simulink model "qdrdacsim"  (R2012b)
settings: Solver=ode45  StartTime=0.0  StopTime=22000  RelTol=1e-3
values from neighbouring files (symbols this model uses):
  T = 95/2    (= 47.5)    [fluxrampdemodsim.m]
undefined symbols (not defined in the file or in its folder): FRA, FRT, pfb_coeff_gen_calc, sfp, V
libraries: xbsIndex_r4 x5295, casper_library_misc x85, xps_library x14, casper_library_delays x12, maddogLibrary x4, simulink x2
(part 12 of 52)

== system qdrdacsim/syncDelay ==
  sim_1 : Inport
  io_delay : xbsIndex_r4/Delay  rst=off  infoeditControl=Selection of Reset will increase slice count due to use of real FFs and instead of SRLs  en=off  latency=0  dbl_ovrd=off  reg_retiming=on  block_type=delay
  qdrdacsim_syncDelay_user_data_out : xbsIndex_r4/Gateway In  gui_display_data_type=Fixed-point  arith_type=Unsigned  n_bits=32  bin_pt=0  preci_type=Single  exp_width=8  frac_width=24  quantization="Round  (unbiased: +/- Inf)"  overflow=Saturate  period=1  dbl_ovrd=off  timing_constraint=None  locs_specified=off  LOCs={}  UseAsADC=off  ADCChannel='1'  inherit_from_input=off  hdl_port=on  block_type=gatewayin
  reint1 : xbsIndex_r4/Reinterpret  force_arith_type=on  arith_type=Unsigned  force_bin_pt=on  bin_pt=0  block_type=reinterpret
  slice_reg : xbsIndex_r4/Slice  nbits=16  boolean_output=off  mode=Lower Bit Location + Width  bit1=0  base1=MSB of Input  bit0=0  base0=LSB of Input  dbl_ovrd=off  block_type=slice
  in_reg : Outport
  wires:
  qdrdacsim_syncDelay_user_data_out/1 -> io_delay/1
  sim_1/1 -> qdrdacsim_syncDelay_user_data_out/1
  io_delay/1 -> slice_reg/1
  slice_reg/1 -> reint1/1
  reint1/1 -> in_reg/1

== system qdrdacsim/txdestip ==
  sim_1 : Inport
  io_delay : xbsIndex_r4/Delay  rst=off  infoeditControl=Selection of Reset will increase slice count due to use of real FFs and instead of SRLs  en=off  latency=0  dbl_ovrd=off  reg_retiming=on  block_type=delay
  qdrdacsim_txdestip_user_data_out : xbsIndex_r4/Gateway In  gui_display_data_type=Fixed-point  arith_type=Unsigned  n_bits=32  bin_pt=0  preci_type=Single  exp_width=8  frac_width=24  quantization="Round  (unbiased: +/- Inf)"  overflow=Saturate  period=1  dbl_ovrd=off  timing_constraint=None  locs_specified=off  LOCs={}  UseAsADC=off  ADCChannel='1'  inherit_from_input=off  hdl_port=on  block_type=gatewayin
  reint1 : xbsIndex_r4/Reinterpret  force_arith_type=on  arith_type=Unsigned  force_bin_pt=on  bin_pt=0  block_type=reinterpret
  slice_reg : xbsIndex_r4/Slice  nbits=32  boolean_output=off  mode=Lower Bit Location + Width  bit1=0  base1=MSB of Input  bit0=0  base0=LSB of Input  dbl_ovrd=off  block_type=slice
  in_reg : Outport
  wires:
  qdrdacsim_txdestip_user_data_out/1 -> io_delay/1
  sim_1/1 -> qdrdacsim_txdestip_user_data_out/1
  io_delay/1 -> slice_reg/1
  slice_reg/1 -> reint1/1
  reint1/1 -> in_reg/1

== system qdrdacsim/txdestport ==
  sim_1 : Inport
  io_delay : xbsIndex_r4/Delay  rst=off  infoeditControl=Selection of Reset will increase slice count due to use of real FFs and instead of SRLs  en=off  latency=0  dbl_ovrd=off  reg_retiming=on  block_type=delay
  qdrdacsim_txdestport_user_data_out : xbsIndex_r4/Gateway In  gui_display_data_type=Fixed-point  arith_type=Unsigned  n_bits=32  bin_pt=0  preci_type=Single  exp_width=8  frac_width=24  quantization="Round  (unbiased: +/- Inf)"  overflow=Saturate  period=1  dbl_ovrd=off  timing_constraint=None  locs_specified=off  LOCs={}  UseAsADC=off  ADCChannel='1'  inherit_from_input=off  hdl_port=on  block_type=gatewayin
  reint1 : xbsIndex_r4/Reinterpret  force_arith_type=on  arith_type=Unsigned  force_bin_pt=on  bin_pt=0  block_type=reinterpret
  slice_reg : xbsIndex_r4/Slice  nbits=16  boolean_output=off  mode=Lower Bit Location + Width  bit1=0  base1=MSB of Input  bit0=0  base0=LSB of Input  dbl_ovrd=off  block_type=slice
  in_reg : Outport
  wires:
  qdrdacsim_txdestport_user_data_out/1 -> io_delay/1
  sim_1/1 -> qdrdacsim_txdestport_user_data_out/1
  io_delay/1 -> slice_reg/1
  slice_reg/1 -> reint1/1
  reint1/1 -> in_reg/1

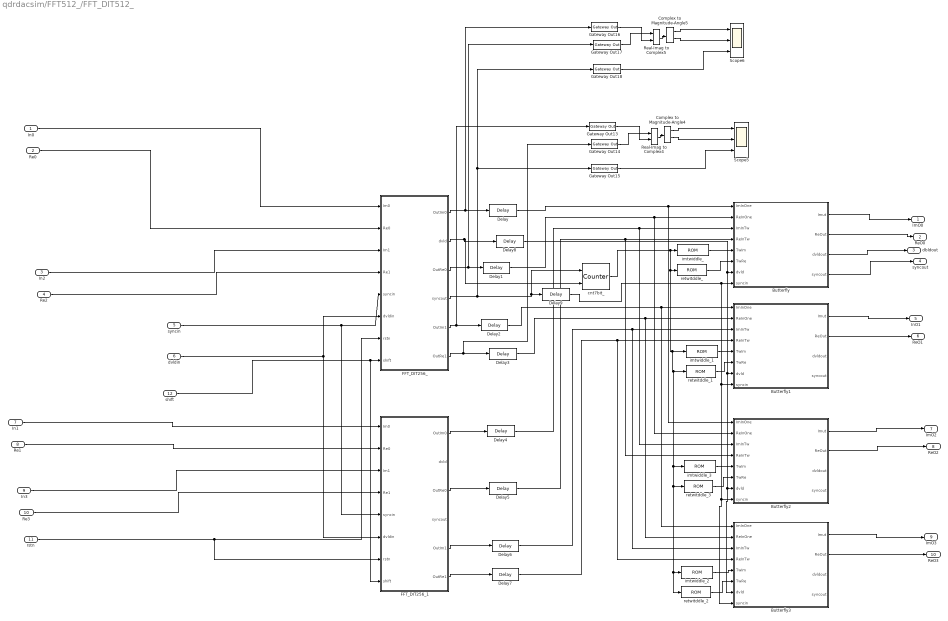
== system qdrdacsim/FFT512_/FFT_DIT512_ ==
  In0 : Inport
  Re0 : Inport  Port=2
  In2 : Inport  Port=3
  Re2 : Inport  Port=4
  syncin : Inport  Port=5
  dvldin : Inport  Port=6
  In1 : Inport  Port=7
  Re1 : Inport  Port=8
  In3 : Inport  Port=9
  Re3 : Inport  Port=10
  rstn : Inport  Port=11
  shift : Inport  Port=12
  Butterfly : Subsystem
  Butterfly1 : Subsystem
  Butterfly2 : Subsystem
  Butterfly3 : Subsystem
  Complex to Magnitude-Angle4 : ComplexToMagnitudeAngle
  Complex to Magnitude-Angle5 : ComplexToMagnitudeAngle
  Delay{,1..9} (10 alike) : xbsIndex_r4/Delay  rst=off  infoeditControl=Selection of Reset will increase slice count due to use of real FFs and instead of SRLs  en=off  latency=1  dbl_ovrd=off  reg_retiming=off  block_type=delay
  FFT_DIT256_ : Subsystem
  FFT_DIT256_1 : Subsystem
  Gateway Out{13..18} (6 alike) : xbsIndex_r4/Gateway Out  inherit_from_input=off  hdl_port=on  timing_constraint=None  locs_specified=off  LOCs={}  UseAsDAC=off  DACChannel='1'  block_type=gatewayout
  Real-Imag to Complex4 : RealImagToComplex
  Real-Imag to Complex5 : RealImagToComplex
  Scope5 : Scope  NumInputPorts=3
      settings: YMin=-5~-5~-5  YMax=5~5~5  SaveName=ScopeData7
  Scope6 : Scope  NumInputPorts=3
      settings: YMin=-5~-5~-5  YMax=5~5~5  SaveName=ScopeData10
  cnt7bit_ : xbsIndex_r4/Counter  cnt_type=Free Running  cnt_to=Inf  operation=Up  start_count=0  cnt_by_val=1  arith_type=Unsigned  n_bits=7  bin_pt=0  load_pin=off  rst=on  en=on  explicit_period=on  period=1  dbl_ovrd=off  use_behavioral_HDL=off  implementation=Fabric  block_type=counter
  imtwiddle_ : xbsIndex_r4/ROM  depth=128  initVector=-sin(2*pi*(0:127)/512)  distributed_mem=Block RAM  rst=off  init_reg=0  en=off  latency=1  gui_display_data_type=Fixed-point  arith_type="Signed  (2's comp)"  n_bits=16  bin_pt=15  preci_type=Single  exp_width=8  frac_width=24  dbl_ovrd=off  optimize=Area  use_rpm=on  block_type=sprom
  imtwiddle_1 : xbsIndex_r4/ROM  depth=128  initVector=-sin(2*pi*(128:255)/512)  distributed_mem=Block RAM  rst=off  init_reg=0  en=off  latency=1  gui_display_data_type=Fixed-point  arith_type="Signed  (2's comp)"  n_bits=16  bin_pt=15  preci_type=Single  exp_width=8  frac_width=24  dbl_ovrd=off  optimize=Area  use_rpm=on  block_type=sprom
  imtwiddle_2 : xbsIndex_r4/ROM  depth=128  initVector=-sin(2*pi*(384:511)/512)  distributed_mem=Block RAM  rst=off  init_reg=0  en=off  latency=1  gui_display_data_type=Fixed-point  arith_type="Signed  (2's comp)"  n_bits=16  bin_pt=15  preci_type=Single  exp_width=8  frac_width=24  dbl_ovrd=off  optimize=Area  use_rpm=on  block_type=sprom
  imtwiddle_3 : xbsIndex_r4/ROM  depth=128  initVector=-sin(2*pi*(256:383)/512)  distributed_mem=Block RAM  rst=off  init_reg=0  en=off  latency=1  gui_display_data_type=Fixed-point  arith_type="Signed  (2's comp)"  n_bits=16  bin_pt=15  preci_type=Single  exp_width=8  frac_width=24  dbl_ovrd=off  optimize=Area  use_rpm=on  block_type=sprom
  retwitddle_ : xbsIndex_r4/ROM  depth=128  initVector=cos(2*pi*(0:127)/512)  distributed_mem=Block RAM  rst=off  init_reg=0  en=off  latency=1  gui_display_data_type=Fixed-point  arith_type="Signed  (2's comp)"  n_bits=16  bin_pt=14  preci_type=Single  exp_width=8  frac_width=24  dbl_ovrd=off  optimize=Area  use_rpm=on  block_type=sprom
  retwitddle_1 : xbsIndex_r4/ROM  depth=128  initVector=cos(2*pi*(128:255)/512)  distributed_mem=Block RAM  rst=off  init_reg=0  en=off  latency=1  gui_display_data_type=Fixed-point  arith_type="Signed  (2's comp)"  n_bits=16  bin_pt=14  preci_type=Single  exp_width=8  frac_width=24  dbl_ovrd=off  optimize=Area  use_rpm=on  block_type=sprom
  retwitddle_2 : xbsIndex_r4/ROM  depth=128  initVector=cos(2*pi*(384:511)/512)  distributed_mem=Block RAM  rst=off  init_reg=0  en=off  latency=1  gui_display_data_type=Fixed-point  arith_type="Signed  (2's comp)"  n_bits=16  bin_pt=14  preci_type=Single  exp_width=8  frac_width=24  dbl_ovrd=off  optimize=Area  use_rpm=on  block_type=sprom
  retwitddle_3 : xbsIndex_r4/ROM  depth=128  initVector=cos(2*pi*(256:383)/512)  distributed_mem=Block RAM  rst=off  init_reg=0  en=off  latency=1  gui_display_data_type=Fixed-point  arith_type="Signed  (2's comp)"  n_bits=16  bin_pt=14  preci_type=Single  exp_width=8  frac_width=24  dbl_ovrd=off  optimize=Area  use_rpm=on  block_type=sprom
  ImO0 : Outport
  ReO0 : Outport  Port=2
  dbldout : Outport  Port=3
  syncout : Outport  Port=4
  InO1 : Outport  Port=5
  ReO1 : Outport  Port=6
  ImO2 : Outport  Port=7
  ReO2 : Outport  Port=8
  ImO3 : Outport  Port=9
  ReO3 : Outport  Port=10
  wires:
  Delay1/1 -> Butterfly2/2(ReInOne), Butterfly/2(ReInOne)
  FFT_DIT256_1/1(OutIm0) -> Delay4/1
  Real-Imag to Complex4/1 -> Complex to Magnitude-Angle4/1
  In1/1 -> FFT_DIT256_1/1(Im0)
  Butterfly1/2(ReOut) -> ReO1/1
  FFT_DIT256_/3(OutRe0) -> Gateway Out17/1, Delay1/1
  FFT_DIT256_/2(dvld) -> Delay8/1, cnt7bit_/2
  Butterfly2/1(Imut) -> ImO2/1
  Complex to Magnitude-Angle5/2 -> Scope6/2
  Delay3/1 -> Butterfly3/2(ReInOne), Butterfly1/2(ReInOne)
  In3/1 -> FFT_DIT256_1/3(Im1)
  retwitddle_1/1 -> Butterfly1/6(TwRe)
  dvldin/1 -> FFT_DIT256_/6(dvldin), FFT_DIT256_1/6(dvldin)
  FFT_DIT256_1/3(OutRe0) -> Delay5/1
  Re3/1 -> FFT_DIT256_1/4(Re1)
  Delay5/1 -> Butterfly2/4(ReInTw), Butterfly/4(ReInTw)
  cnt7bit_/1 -> retwitddle_2/1, imtwiddle_2/1, retwitddle_3/1, imtwiddle_3/1, retwitddle_1/1, imtwiddle_1/1, retwitddle_/1, imtwiddle_/1
  Gateway Out18/1 -> Scope6/3
  Delay6/1 -> Butterfly3/3(ImInTw), Butterfly1/3(ImInTw)
  imtwiddle_2/1 -> Butterfly3/5(TwIm)
  Delay4/1 -> Butterfly2/3(ImInTw), Butterfly/3(ImInTw)
  Gateway Out13/1 -> Real-Imag to Complex4/2
  retwitddle_2/1 -> Butterfly3/6(TwRe)
  Re2/1 -> FFT_DIT256_/4(Re1)
  Gateway Out16/1 -> Real-Imag to Complex5/2
  Re0/1 -> FFT_DIT256_/2(Re0)
  Butterfly/3(dvldout) -> dbldout/1
  Gateway Out17/1 -> Real-Imag to Complex5/1
  Delay/1 -> Butterfly2/1(ImInOne), Butterfly/1(ImInOne)
  Butterfly3/1(Imut) -> ImO3/1
  retwitddle_3/1 -> Butterfly2/6(TwRe)
  imtwiddle_/1 -> Butterfly/5(TwIm)
  imtwiddle_3/1 -> Butterfly2/5(TwIm)
  FFT_DIT256_/1(OutIm0) -> Gateway Out16/1, Delay/1
  Butterfly3/2(ReOut) -> ReO3/1
  Butterfly/1(Imut) -> ImO0/1
  Butterfly/2(ReOut) -> ReO0/1
  FFT_DIT256_1/6(OutRe1) -> Delay7/1
  Delay9/1 -> Butterfly3/8(syncin), Butterfly2/8(syncin), Butterfly1/8(syncin), Butterfly/8(syncin)
  FFT_DIT256_1/5(OutIm1) -> Delay6/1
  Butterfly1/1(Imut) -> InO1/1
  imtwiddle_1/1 -> Butterfly1/5(TwIm)
  Re1/1 -> FFT_DIT256_1/2(Re0)
  Butterfly/4(syncout) -> syncout/1
  FFT_DIT256_/6(OutRe1) -> Gateway Out14/1, Delay3/1
  In0/1 -> FFT_DIT256_/1(Im0)
  Gateway Out14/1 -> Real-Imag to Complex4/1
  Delay7/1 -> Butterfly3/4(ReInTw), Butterfly1/4(ReInTw)
  Butterfly2/2(ReOut) -> ReO2/1
  FFT_DIT256_/4(syncout) -> Gateway Out15/1, Gateway Out18/1, Delay9/1, cnt7bit_/1
  Complex to Magnitude-Angle5/1 -> Scope6/1
  Delay8/1 -> Butterfly3/7(dvld), Butterfly2/7(dvld), Butterfly1/7(dvld), Butterfly/7(dvld)
  FFT_DIT256_/5(OutIm1) -> Gateway Out13/1, Delay2/1
  Real-Imag to Complex5/1 -> Complex to Magnitude-Angle5/1
  retwitddle_/1 -> Butterfly/6(TwRe)
  Complex to Magnitude-Angle4/2 -> Scope5/2
  In2/1 -> FFT_DIT256_/3(Im1)
  Gateway Out15/1 -> Scope5/3
  syncin/1 -> FFT_DIT256_1/5(syncin), FFT_DIT256_/5(syncin)
  Complex to Magnitude-Angle4/1 -> Scope5/1
  Delay2/1 -> Butterfly3/1(ImInOne), Butterfly1/1(ImInOne)
  rstn/1 -> FFT_DIT256_1/7(rstn), FFT_DIT256_/7(rstn)
  shift/1 -> FFT_DIT256_1/8(shift), FFT_DIT256_/8(shift)

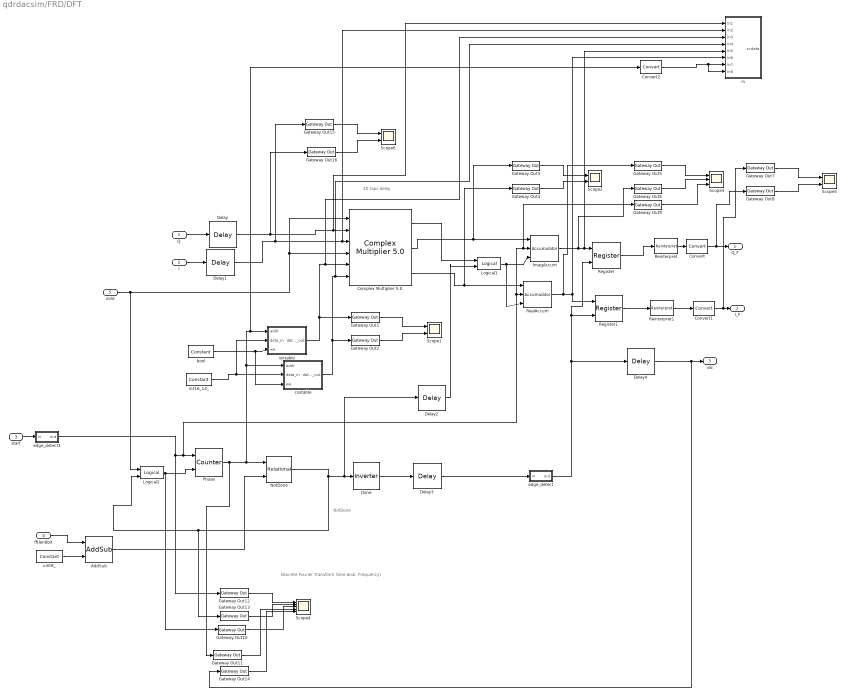
== system qdrdacsim/FRD/DFT ==
  note: 40 taps delay
  note: Discrete Fourier Transform
      | (One Anal. Frequency)
  note: NotDone
  Q : Inport
  I : Inport  Port=2
  start : Inport  Port=3
  fftlen8bit : Inport  Port=4
  dvld : Inport  Port=5
  AddSub : xbsIndex_r4/AddSub  mode=Subtraction  use_carryin=off  use_carryout=off  en=off  latency=0  precision=Full  arith_type=Unsigned  n_bits=16  bin_pt=14  quantization=Truncate  overflow=Wrap  dbl_ovrd=off  use_behavioral_HDL=off  hw_selection=Fabric  pipelined=off  block_type=addsub
  "Complex Multiplier 5.0 " : xbsIndex_r4/Complex Multiplier 5.0   hasatlast=off  hasatuser=off  atuserwidth=1  hasbtlast=off  hasbtuser=off  btuserwidth=1  multtype=Use_Mults  optimizegoal=Resources  flowcontrol=NonBlocking  outputwidth=20  roundmode=Truncate  hasctrltlast=off  hasctrltuser=off  ctrltuserwidth=1  outtlastbehv=Null  latencyconfig=Manual  minimumlatency=40  aclken=off  aresetn=off  trim_axipin_name=on  aportwidth=63  bportwidth=63  ip_name=Complex Multiplier  ip_version=5.0  dsptool_ready=true  ipcore_usecache=true  ipcore_useipmodelcache=true  ipcore_verbose=false  ipcore_latency_parameter='minimumlatency'  wrapper_available=true  port_translation_map={ 'aclken' => 'en', 'aresetn' => 'rst'}  structural_sim=false  block_type=cmpy_v5_0
  Convert : xbsIndex_r4/Convert  gui_display_data_type=Fixed-point  arith_type="Signed  (2's comp)"  n_bits=16  bin_pt=14  float_type=Single  exp_bits=8  fraction_bits=24  quantization=Truncate  overflow=Wrap  en=off  latency=0  dbl_ovrd=off  pipeline=off  block_type=convert
  Convert1 : xbsIndex_r4/Convert  gui_display_data_type=Fixed-point  arith_type="Signed  (2's comp)"  n_bits=16  bin_pt=14  float_type=Single  exp_bits=8  fraction_bits=24  quantization=Truncate  overflow=Wrap  en=off  latency=0  dbl_ovrd=off  pipeline=off  block_type=convert
  Convert2 : xbsIndex_r4/Convert  gui_display_data_type=Fixed-point  arith_type=Unsigned  n_bits=16  bin_pt=0  float_type=Single  exp_bits=8  fraction_bits=24  quantization=Truncate  overflow=Wrap  en=off  latency=0  dbl_ovrd=off  pipeline=off  block_type=convert
  Delay : xbsIndex_r4/Delay  rst=off  infoeditControl=Selection of Reset will increase slice count due to use of real FFs and instead of SRLs  en=off  latency=1  dbl_ovrd=off  reg_retiming=off  block_type=delay
  Delay1 : xbsIndex_r4/Delay  rst=off  infoeditControl=Selection of Reset will increase slice count due to use of real FFs and instead of SRLs  en=off  latency=1  dbl_ovrd=off  reg_retiming=off  block_type=delay
  Delay2 : xbsIndex_r4/Delay  rst=off  infoeditControl=Selection of Reset will increase slice count due to use of real FFs and instead of SRLs  en=off  latency=41  dbl_ovrd=off  reg_retiming=off  block_type=delay
  Delay3 : xbsIndex_r4/Delay  rst=off  infoeditControl=Selection of Reset will increase slice count due to use of real FFs and instead of SRLs  en=off  latency=42  dbl_ovrd=off  reg_retiming=off  block_type=delay
  Delay4 : xbsIndex_r4/Delay  rst=off  infoeditControl=Selection of Reset will increase slice count due to use of real FFs and instead of SRLs  en=off  latency=1  dbl_ovrd=off  reg_retiming=off  block_type=delay
  Done : xbsIndex_r4/Inverter  en=off  latency=0  dbl_ovrd=off  block_type=inv
  Gateway Out{1..16} (16 alike) : xbsIndex_r4/Gateway Out  inherit_from_input=off  hdl_port=on  timing_constraint=None  locs_specified=off  LOCs={}  UseAsDAC=off  DACChannel='1'  block_type=gatewayout
  ImagAccum : xbsIndex_r4/Accumulator  operation=Add  n_bits=24  overflow=Wrap  scale=1  rst=on  infoeditControl=reset for floating point data type must be asserted for a minimum of 2 cycles  hasbypass=off  en=on  latency=0  dbl_ovrd=off  msb_inp=100  msb=100  lsb=-100  use_behavioral_HDL=on  implementation=Fabric  block_type=accum
  Logical1 : xbsIndex_r4/Logical  logical_function=AND  inputs=2  en=off  latency=0  precision=Full  arith_type=Unsigned  n_bits=16  bin_pt=0  align_bp=on  dbl_ovrd=off  block_type=logical
  Logical2 : xbsIndex_r4/Logical  logical_function=AND  inputs=2  en=off  latency=0  precision=Full  arith_type=Unsigned  n_bits=16  bin_pt=0  align_bp=on  dbl_ovrd=off  block_type=logical
  NotDone : xbsIndex_r4/Relational  mode=a!=b  en=off  latency=0  dbl_ovrd=off  block_type=relational
  Phase : xbsIndex_r4/Counter  cnt_type=Free Running  cnt_to=Inf  operation=Up  start_count=0  cnt_by_val=1  arith_type=Unsigned  n_bits=8  bin_pt=0  load_pin=off  rst=on  en=on  explicit_period=on  period=1  dbl_ovrd=off  use_behavioral_HDL=off  implementation=Fabric  block_type=counter
  RealAccum : xbsIndex_r4/Accumulator  operation=Add  n_bits=24  overflow=Wrap  scale=1  rst=on  infoeditControl=reset for floating point data type must be asserted for a minimum of 2 cycles  hasbypass=off  en=on  latency=0  dbl_ovrd=off  msb_inp=100  msb=100  lsb=-100  use_behavioral_HDL=on  implementation=Fabric  block_type=accum
  Register : xbsIndex_r4/Register  init=0  rst=off  en=on  dbl_ovrd=off  block_type=register
  Register1 : xbsIndex_r4/Register  init=0  rst=off  en=on  dbl_ovrd=off  block_type=register
  Reinterpret : xbsIndex_r4/Reinterpret  force_arith_type=on  arith_type="Signed  (2's comp)"  force_bin_pt=on  bin_pt=18  block_type=reinterpret
  Reinterpret1 : xbsIndex_r4/Reinterpret  force_arith_type=on  arith_type="Signed  (2's comp)"  force_bin_pt=on  bin_pt=18  block_type=reinterpret
  Scope{1..2,5..6} (4 alike) : Scope  NumInputPorts=2
      Scope1 settings: YMin=-5~-5  YMax=5~5  SaveName=ScopeData7  MaxDataPoints=1800
      Scope2 settings: YMin=-5~-5  YMax=5~5  SaveName=ScopeData8  MaxDataPoints=1800
      Scope5 settings: YMin=-5~-5  YMax=5~5  SaveName=ScopeData10  MaxDataPoints=1800
      Scope6 settings: YMin=-5~-5  YMax=5~5  MaxDataPoints=1800
  Scope3 : Scope  NumInputPorts=3
      settings: YMin=-5~-5~-5  YMax=5~5~5  SaveName=ScopeData9  MaxDataPoints=1800
  Scope4 : Scope  NumInputPorts=5
      settings: YMin=-5~-5~-5~-5~-5  YMax=5~5~5~5~5  SaveName=ScopeData6  MaxDataPoints=1800
  bool : xbsIndex_r4/Constant  const=0  gui_display_data_type=Boolean  arith_type=Boolean  n_bits=16  bin_pt=14  preci_type=Single  exp_width=8  frac_width=24  explicit_period=on  period=1  equ=P=C  opselect=C  inp2=PCIN>>17  opr=+  inp1=P  carry=CIN  dbl_ovrd=off  block_type=constant
  costable : Subsystem  Tag=xps:bram  AncestorBlock=xps_library/Shared BRAM  mask{arith_type=Signed  (2's comp), addr_width=11, data_width=16, reg_prim_output=off, reg_core_output=off, optimization=Minimum_Area, data_bin_pt=14, init_vals=cos(3*2*pi*(0:89)/90) .* hamming(90)', sample_rate=1}
      mask prompts: arith_type "Output Data Type"; addr_width "Address width"; data_width "Data Width"; reg_prim_output "Register Primitive Output"; reg_core_output "Register Core Output"; data_bin_pt "Data Binary Point"; init_vals "Initial values (simulation only)"; sample_rate "Sample rate"
      mask init:
      | shared_bram_mask;
      mask TypeOptions arith_type: Unsigned | Signed  (2's comp)
      mask TypeOptions data_width: 8 | 16 | 32 | 64 | 128
      mask TypeOptions optimization: Minimum_Area | Low_Power
  edge_detect : Subsystem  AncestorBlock=casper_library_misc/edge_detect  mask(edge_detect){edge=Rising, polarity=Active High, x_in=[0 0.08 0.08 0.16 0.16 0.24 0.24 0.32 0.32 0.4], y_in=[-1 -1  1  1  1  1  1  1  1  1], x_out=[0.6 0.68 0.68 0.76 0.76 0.84 0.84 0.92 0.92 1], y_out=[-1 -1  1  1 -1 -1 -1 -1 -1 -1]}
      mask prompts: edge "Edge Type"; polarity "Output Polarity"; x_in "Input X Positions"; y_in "Input Y Positions"; x_out "Output X Positions"; y_out "Output Y Positions"
      mask help: Output is active for one-cycle after each edge of the specified type (i.e. rising, falling or both).
      mask init: same as qdrdacsim/edge_detect
      settings: AttributesFormatString=|
      | rising edges
      | active high
      mask Help: Output is active for one-cycle after each edge of the specified type (i.e. rising, falling, or both).  Latency is zero.
      mask TypeOptions edge: Rising | Falling | Both
      mask TypeOptions polarity: Active High | Active Low
      mask Display:
      | plot(x_in_num,0.5+y_in_num*0.2);
      | plot(x_out_num,0.5+y_out_num*0.2);
  edge_detect1 : Subsystem  AncestorBlock=casper_library_misc/edge_detect  mask(edge_detect){edge=Rising, polarity=Active High, x_in=[0 0.08 0.08 0.16 0.16 0.24 0.24 0.32 0.32 0.4], y_in=[-1 -1  1  1  1  1  1  1  1  1], x_out=[0.6 0.68 0.68 0.76 0.76 0.84 0.84 0.92 0.92 1], y_out=[-1 -1  1  1 -1 -1 -1 -1 -1 -1]}
      mask prompts: edge "Edge Type"; polarity "Output Polarity"; x_in "Input X Positions"; y_in "Input Y Positions"; x_out "Output X Positions"; y_out "Output Y Positions"
      mask help: Output is active for one-cycle after each edge of the specified type (i.e. rising, falling or both).
      mask init: same as qdrdacsim/edge_detect
      settings: AttributesFormatString=|
      | rising edges
      | active high
      mask Help: Output is active for one-cycle after each edge of the specified type (i.e. rising, falling, or both).  Latency is zero.
      mask TypeOptions edge: Rising | Falling | Both
      mask TypeOptions polarity: Active High | Active Low
      mask Display:
      | plot(x_in_num,0.5+y_in_num*0.2);
      | plot(x_out_num,0.5+y_out_num*0.2);
  int16_14_ : xbsIndex_r4/Constant  const=0  gui_display_data_type=Fixed-point  arith_type=Signed (2's comp)  n_bits=16  bin_pt=14  preci_type=Single  exp_width=8  frac_width=24  explicit_period=on  period=1  equ=P=C  opselect=C  inp2=PCIN>>17  opr=+  inp1=P  carry=CIN  dbl_ovrd=off  block_type=constant
  rs : Subsystem
  sintable : Subsystem  Tag=xps:bram  AncestorBlock=xps_library/Shared BRAM  mask{arith_type=Signed  (2's comp), addr_width=11, data_width=16, reg_prim_output=off, reg_core_output=off, optimization=Minimum_Area, data_bin_pt=14, init_vals=(-sin(3*2*pi*(0:89)/90)) .* hamming(90)', sample_rate=1}
      mask prompts: arith_type "Output Data Type"; addr_width "Address width"; data_width "Data Width"; reg_prim_output "Register Primitive Output"; reg_core_output "Register Core Output"; data_bin_pt "Data Binary Point"; init_vals "Initial values (simulation only)"; sample_rate "Sample rate"
      mask init:
      | shared_bram_mask;
      mask TypeOptions arith_type: Unsigned | Signed  (2's comp)
      mask TypeOptions data_width: 8 | 16 | 32 | 64 | 128
      mask TypeOptions optimization: Minimum_Area | Low_Power
  uint8_ : xbsIndex_r4/Constant  const=1  gui_display_data_type=Fixed-point  arith_type=Unsigned  n_bits=8  bin_pt=0  preci_type=Single  exp_width=8  frac_width=24  explicit_period=on  period=1  equ=P=C  opselect=C  inp2=PCIN>>17  opr=+  inp1=P  carry=CIN  dbl_ovrd=off  block_type=constant
  Q_F : Outport
  I_F : Outport  Port=2
  vld : Outport  Port=3
  wires:
  "Complex Multiplier 5.0 "/2 -> Gateway Out3/1, ImagAccum/1
  I/1 -> Delay1/1
  Phase/1 -> Gateway Out11/1, costable/1(addr), Convert2/1, sintable/1(addr), NotDone/1
  NotDone/1 -> Gateway Out13/1, Logical2/2, Delay2/1, Done/1
  Q/1 -> Delay/1
  costable/1(data_out) -> Gateway Out2/1, rs/4(In4), "Complex Multiplier 5.0 "/6
  Done/1 -> Delay3/1
  sintable/1(data_out) -> Gateway Out1/1, rs/3(In3), "Complex Multiplier 5.0 "/5
  Register1/1 -> Reinterpret1/1
  Register/1 -> Reinterpret/1
  ImagAccum/1 -> Gateway Out6/1, rs/5(In5), Register/1
  RealAccum/1 -> Gateway Out5/1, rs/6(In6), Register1/1
  edge_detect/1(out) -> Delay4/1, Register/2, Register1/2
  Delay/1 -> Gateway Out16/1, rs/1(In1), "Complex Multiplier 5.0 "/2
  Delay1/1 -> Gateway Out15/1, rs/2(In2), "Complex Multiplier 5.0 "/3
  edge_detect1/1(out) -> Gateway Out12/1, Gateway Out9/1, ImagAccum/2, RealAccum/2, Phase/1
  Delay3/1 -> edge_detect/1(in)
  "Complex Multiplier 5.0 "/3 -> Gateway Out4/1, RealAccum/1
  Reinterpret/1 -> Convert/1
  Reinterpret1/1 -> Convert1/1
  Convert/1 -> Gateway Out8/1, Q_F/1
  Convert1/1 -> Gateway Out7/1, I_F/1
  Gateway Out13/1 -> Scope4/2
  Gateway Out12/1 -> Scope4/1
  Gateway Out2/1 -> Scope1/2
  Gateway Out1/1 -> Scope1/1
  Gateway Out4/1 -> Scope2/2
  Gateway Out3/1 -> Scope2/1
  Gateway Out6/1 -> Scope3/2
  Gateway Out5/1 -> Scope3/1
  Gateway Out8/1 -> Scope5/2
  Gateway Out7/1 -> Scope5/1
  Gateway Out9/1 -> Scope3/3
  start/1 -> edge_detect1/1(in)
  uint8_/1 -> AddSub/2
  fftlen8bit/1 -> AddSub/1
  AddSub/1 -> NotDone/2
  dvld/1 -> Logical2/1, "Complex Multiplier 5.0 "/4, "Complex Multiplier 5.0 "/1
  Delay2/1 -> Logical1/2
  "Complex Multiplier 5.0 "/1 -> Logical1/1
  Logical1/1 -> RealAccum/3, ImagAccum/3
  Logical2/1 -> Gateway Out10/1, Phase/2
  Gateway Out10/1 -> Scope4/3
  Gateway Out11/1 -> Scope4/4
  Gateway Out14/1 -> Scope4/5
  Gateway Out16/1 -> Scope6/2
  Gateway Out15/1 -> Scope6/1
  Delay4/1 -> Gateway Out14/1, vld/1
  bool/1 -> costable/3(we), sintable/3(we)
  int16_14_/1 -> sintable/2(data_in), costable/2(data_in)
  Convert2/1 -> rs/8(In8), rs/7(In7)

== system qdrdacsim/FRD/PhaseUnwrap ==
  note: FixPosJump
  note: Fix Neg Jup
  note: Determine If Phase Jump
  note: Calculate if we have Phase Jump
      | by comparing derivative of phase wrt time
      | to pi and -pi.
  note: Perform Phase Unwrap by adding
      | 0 , 2pi or -2pi
  note: State 0 : Add 0 to phase
      | Sate 1: Add 2pi to phase
      | State 2: Add -2pi to phase
      | State 3: Error
  note: Phase Unwrap
  note: State Machine Next State
  note: Error Flag Output
  note: Phase Addend:
      | 0.0, 2pi or -2pi
  note: Calc. Unwrapped
      | Phase
  note: How the muxes work
      |
      | always @(posedge clk)
      | //NextStae Mux
      | switch State:
      | {
      | 	0: //add 0 to phase
      | 		switch {negjmp, posjmp}
      | 		{
      | 			0: state<=0; break;
      | 			1: state,=1;break
      | 			2:state <=2; break
      | 			3:state <=3;
      | 		}
      | 		break
      |
      | 	1: // add
  Phase : Inport
  Rst : Inport  Port=2
  vld_in : Inport  Port=3
  mag_in : Inport  Port=4
  AddSub : xbsIndex_r4/AddSub  mode=Addition  use_carryin=off  use_carryout=off  en=off  latency=1  precision=User Defined  arith_type="Signed  (2's comp)"  n_bits=16  bin_pt=13  quantization=Truncate  overflow=Wrap  dbl_ovrd=off  use_behavioral_HDL=off  hw_selection=Fabric  pipelined=off  block_type=addsub
  Concat : xbsIndex_r4/Concat  num_inputs=2  dbl_ovrd=off  block_type=concat
  Constant : xbsIndex_r4/Constant  const=0  gui_display_data_type=Fixed-point  arith_type=Signed (2's comp)  n_bits=16  bin_pt=13  preci_type=Single  exp_width=8  frac_width=24  explicit_period=on  period=1  equ=P=C  opselect=C  inp2=PCIN>>17  opr=+  inp1=P  carry=CIN  dbl_ovrd=off  block_type=constant
  Constant1 : xbsIndex_r4/Constant  const=-2  gui_display_data_type=Fixed-point  arith_type=Signed (2's comp)  n_bits=16  bin_pt=13  preci_type=Single  exp_width=8  frac_width=24  explicit_period=on  period=1  equ=P=C  opselect=C  inp2=PCIN>>17  opr=+  inp1=P  carry=CIN  dbl_ovrd=off  block_type=constant
  Constant10 : xbsIndex_r4/Constant  const=0  gui_display_data_type=Fixed-point  arith_type=Unsigned  n_bits=2  bin_pt=0  preci_type=Single  exp_width=8  frac_width=24  explicit_period=on  period=1  equ=P=C  opselect=C  inp2=PCIN>>17  opr=+  inp1=P  carry=CIN  dbl_ovrd=off  block_type=constant
  Constant{8,11..13,15,17} (6 alike) : xbsIndex_r4/Constant  const=3  gui_display_data_type=Fixed-point  arith_type=Unsigned  n_bits=2  bin_pt=0  preci_type=Single  exp_width=8  frac_width=24  explicit_period=on  period=1  equ=P=C  opselect=C  inp2=PCIN>>17  opr=+  inp1=P  carry=CIN  dbl_ovrd=off  block_type=constant
  Constant14 : xbsIndex_r4/Constant  const=0  gui_display_data_type=Fixed-point  arith_type=Unsigned  n_bits=2  bin_pt=0  preci_type=Single  exp_width=8  frac_width=24  explicit_period=on  period=1  equ=P=C  opselect=C  inp2=PCIN>>17  opr=+  inp1=P  carry=CIN  dbl_ovrd=off  block_type=constant
  Constant16 : xbsIndex_r4/Constant  const=2  gui_display_data_type=Fixed-point  arith_type=Unsigned  n_bits=2  bin_pt=0  preci_type=Single  exp_width=8  frac_width=24  explicit_period=on  period=1  equ=P=C  opselect=C  inp2=PCIN>>17  opr=+  inp1=P  carry=CIN  dbl_ovrd=off  block_type=constant
  Constant18 : xbsIndex_r4/Constant  const=0  gui_display_data_type=Boolean  arith_type=Boolean  n_bits=2  bin_pt=0  preci_type=Single  exp_width=8  frac_width=24  explicit_period=on  period=1  equ=P=C  opselect=C  inp2=PCIN>>17  opr=+  inp1=P  carry=CIN  dbl_ovrd=off  block_type=constant
  Constant19 : xbsIndex_r4/Constant  const=1  gui_display_data_type=Boolean  arith_type=Boolean  n_bits=2  bin_pt=0  preci_type=Single  exp_width=8  frac_width=24  explicit_period=on  period=1  equ=P=C  opselect=C  inp2=PCIN>>17  opr=+  inp1=P  carry=CIN  dbl_ovrd=off  block_type=constant
  Constant2 : xbsIndex_r4/Constant  const=2  gui_display_data_type=Fixed-point  arith_type=Signed (2's comp)  n_bits=16  bin_pt=13  preci_type=Single  exp_width=8  frac_width=24  explicit_period=on  period=1  equ=P=C  opselect=C  inp2=PCIN>>17  opr=+  inp1=P  carry=CIN  dbl_ovrd=off  block_type=constant
  Constant3 : xbsIndex_r4/Constant  const=-1  gui_display_data_type=Fixed-point  arith_type=Signed (2's comp)  n_bits=16  bin_pt=13  preci_type=Single  exp_width=8  frac_width=24  explicit_period=on  period=1  equ=P=C  opselect=C  inp2=PCIN>>17  opr=+  inp1=P  carry=CIN  dbl_ovrd=off  block_type=constant
  Constant4 : xbsIndex_r4/Constant  const=1.0  gui_display_data_type=Fixed-point  arith_type=Signed (2's comp)  n_bits=16  bin_pt=13  preci_type=Single  exp_width=8  frac_width=24  explicit_period=on  period=1  equ=P=C  opselect=C  inp2=PCIN>>17  opr=+  inp1=P  carry=CIN  dbl_ovrd=off  block_type=constant
  Constant5 : xbsIndex_r4/Constant  const=0  gui_display_data_type=Fixed-point  arith_type=Unsigned  n_bits=2  bin_pt=0  preci_type=Single  exp_width=8  frac_width=24  explicit_period=on  period=1  equ=P=C  opselect=C  inp2=PCIN>>17  opr=+  inp1=P  carry=CIN  dbl_ovrd=off  block_type=constant
  Constant6 : xbsIndex_r4/Constant  const=2  gui_display_data_type=Fixed-point  arith_type=Unsigned  n_bits=2  bin_pt=0  preci_type=Single  exp_width=8  frac_width=24  explicit_period=on  period=1  equ=P=C  opselect=C  inp2=PCIN>>17  opr=+  inp1=P  carry=CIN  dbl_ovrd=off  block_type=constant
  Constant7 : xbsIndex_r4/Constant  const=1  gui_display_data_type=Fixed-point  arith_type=Unsigned  n_bits=2  bin_pt=0  preci_type=Single  exp_width=8  frac_width=24  explicit_period=on  period=1  equ=P=C  opselect=C  inp2=PCIN>>17  opr=+  inp1=P  carry=CIN  dbl_ovrd=off  block_type=constant
  Constant9 : xbsIndex_r4/Constant  const=1  gui_display_data_type=Fixed-point  arith_type=Unsigned  n_bits=2  bin_pt=0  preci_type=Single  exp_width=8  frac_width=24  explicit_period=on  period=1  equ=P=C  opselect=C  inp2=PCIN>>17  opr=+  inp1=P  carry=CIN  dbl_ovrd=off  block_type=constant
  Delay : xbsIndex_r4/Delay  rst=off  infoeditControl=Selection of Reset will increase slice count due to use of real FFs and instead of SRLs  en=off  latency=1  dbl_ovrd=off  reg_retiming=off  block_type=delay
  DiffPhase : xbsIndex_r4/AddSub  mode=Subtraction  use_carryin=off  use_carryout=off  en=off  latency=0  precision=Full  arith_type=Unsigned  n_bits=16  bin_pt=14  quantization=Truncate  overflow=Wrap  dbl_ovrd=off  use_behavioral_HDL=off  hw_selection=Fabric  pipelined=off  block_type=addsub
  ErrorOutput : xbsIndex_r4/Mux  inputs=4  en=off  latency=0  precision=Full  arith_type=Unsigned  n_bits=16  bin_pt=14  quantization=Truncate  overflow=Wrap  dbl_ovrd=off  block_type=mux
  Gateway Out{1..6} (6 alike) : xbsIndex_r4/Gateway Out  inherit_from_input=off  hdl_port=on  timing_constraint=None  locs_specified=off  LOCs={}  UseAsDAC=off  DACChannel='1'  block_type=gatewayout
  NegativeJum : xbsIndex_r4/Relational  mode=a>b  en=off  latency=0  dbl_ovrd=off  block_type=relational
  NextState : xbsIndex_r4/Mux  inputs=4  en=off  latency=0  precision=Full  arith_type=Unsigned  n_bits=16  bin_pt=14  quantization=Truncate  overflow=Wrap  dbl_ovrd=off  block_type=mux
  PhaseAddend : xbsIndex_r4/Mux  inputs=4  en=off  latency=0  precision=Full  arith_type=Unsigned  n_bits=16  bin_pt=14  quantization=Truncate  overflow=Wrap  dbl_ovrd=off  block_type=mux
  PositiveJump : xbsIndex_r4/Relational  mode=a<b  en=off  latency=0  dbl_ovrd=off  block_type=relational
  Scope : Scope  NumInputPorts=2
      settings: YMin=-5~-5  YMax=5~5  SaveName=ScopeData11  MaxDataPoints=1800
  Scope1 : Scope  NumInputPorts=2
      settings: YMin=-5~-5  YMax=5~5  SaveName=ScopeData12  MaxDataPoints=1800
  Scope2 : Scope  NumInputPorts=2
      settings: YMin=-5~-5  YMax=5~5  SaveName=ScopeData13  MaxDataPoints=1800
  State : xbsIndex_r4/Register  init=0  rst=on  en=off  dbl_ovrd=off  block_type=register
  StateNext0 : xbsIndex_r4/Mux  inputs=4  en=off  latency=0  precision=Full  arith_type=Unsigned  n_bits=16  bin_pt=14  quantization=Truncate  overflow=Wrap  dbl_ovrd=off  block_type=mux
  StateNext1 : xbsIndex_r4/Mux  inputs=4  en=off  latency=0  precision=Full  arith_type=Unsigned  n_bits=16  bin_pt=14  quantization=Truncate  overflow=Wrap  dbl_ovrd=off  block_type=mux
  StateNext2 : xbsIndex_r4/Mux  inputs=4  en=off  latency=0  precision=Full  arith_type=Unsigned  n_bits=16  bin_pt=14  quantization=Truncate  overflow=Wrap  dbl_ovrd=off  block_type=mux
  Wait_for_FSM : xbsIndex_r4/Delay  rst=off  infoeditControl=Selection of Reset will increase slice count due to use of real FFs and instead of SRLs  en=off  latency=1  dbl_ovrd=off  reg_retiming=off  block_type=delay
  Wait_for_FSM1 : xbsIndex_r4/Delay  rst=off  infoeditControl=Selection of Reset will increase slice count due to use of real FFs and instead of SRLs  en=off  latency=3  dbl_ovrd=off  reg_retiming=off  block_type=delay
  Wait_for_FSM2 : xbsIndex_r4/Delay  rst=off  infoeditControl=Selection of Reset will increase slice count due to use of real FFs and instead of SRLs  en=off  latency=3  dbl_ovrd=off  reg_retiming=off  block_type=delay
  UwrPhase : Outport
  Err : Outport  Port=2
  vld_out : Outport  Port=3
  mag_out : Outport  Port=4
  wires:
  Delay/1 -> DiffPhase/1
  Constant19/1 -> ErrorOutput/5
  NextState/1 -> State/1
  StateNext1/1 -> NextState/3
  Constant9/1 -> StateNext1/2
  PositiveJump/1 -> Gateway Out5/1, Concat/2
  Constant13/1 -> StateNext2/4
  Constant15/1 -> StateNext2/5
  DiffPhase/1 -> PositiveJump/1, NegativeJum/1
  State/1 -> Gateway Out1/1, ErrorOutput/1, PhaseAddend/1, NextState/1
  Constant10/1 -> StateNext1/4
  Constant11/1 -> StateNext1/3
  PhaseAddend/1 -> Gateway Out2/1, AddSub/2
  Constant2/1 -> PhaseAddend/4
  Concat/1 -> StateNext1/1, StateNext0/1, StateNext2/1
  Constant5/1 -> StateNext0/2
  ErrorOutput/1 -> Err/1
  Rst/1 -> State/2
  Constant17/1 -> NextState/5
  AddSub/1 -> Gateway Out6/1, UwrPhase/1
  Constant/1 -> PhaseAddend/5, PhaseAddend/2
  Phase/1 -> DiffPhase/2, Delay/1, Wait_for_FSM/1
  Constant4/1 -> NegativeJum/2
  StateNext0/1 -> NextState/2
  Constant16/1 -> StateNext2/2
  Constant14/1 -> StateNext2/3
  Constant12/1 -> StateNext1/5
  Wait_for_FSM/1 -> Gateway Out3/1, AddSub/1
  Constant8/1 -> StateNext0/5
  Constant7/1 -> StateNext0/3
  Constant18/1 -> ErrorOutput/4, ErrorOutput/3, ErrorOutput/2
  Constant6/1 -> StateNext0/4
  StateNext2/1 -> NextState/4
  NegativeJum/1 -> Gateway Out4/1, Concat/1
  Constant3/1 -> PositiveJump/2
  Constant1/1 -> PhaseAddend/3
  vld_in/1 -> Wait_for_FSM1/1
  Wait_for_FSM1/1 -> vld_out/1
  Wait_for_FSM2/1 -> mag_out/1
  mag_in/1 -> Wait_for_FSM2/1
  Gateway Out5/1 -> Scope/2
  Gateway Out4/1 -> Scope/1
  Gateway Out2/1 -> Scope1/2
  Gateway Out1/1 -> Scope1/1
  Gateway Out6/1 -> Scope2/2
  Gateway Out3/1 -> Scope2/1

== system qdrdacsim/FRD/TranslateIQ ==
  note: Translation in IQ Plane
  Q : Inport
  I : Inport  Port=2
  vld_in : Inport  Port=3
  Delay : xbsIndex_r4/Delay  rst=off  infoeditControl=Selection of Reset will increase slice count due to use of real FFs and instead of SRLs  en=off  latency=1  dbl_ovrd=off  reg_retiming=off  block_type=delay
  trot_xoffset : xbsIndex_r4/Constant  const=0.0  gui_display_data_type=Fixed-point  arith_type=Signed (2's comp)  n_bits=16  bin_pt=14  preci_type=Single  exp_width=8  frac_width=24  explicit_period=off  period=1  equ=P=C  opselect=C  inp2=PCIN>>17  opr=+  inp1=P  carry=CIN  dbl_ovrd=off  block_type=constant
  trot_yoffset : xbsIndex_r4/Constant  const=0.0  gui_display_data_type=Fixed-point  arith_type=Signed (2's comp)  n_bits=16  bin_pt=14  preci_type=Single  exp_width=8  frac_width=24  explicit_period=off  period=1  equ=P=C  opselect=C  inp2=PCIN>>17  opr=+  inp1=P  carry=CIN  dbl_ovrd=off  block_type=constant
  trotimag : xbsIndex_r4/AddSub  mode=Addition  use_carryin=off  use_carryout=off  en=off  latency=1  precision=User Defined  arith_type="Signed  (2's comp)"  n_bits=16  bin_pt=14  quantization=Truncate  overflow=Wrap  dbl_ovrd=off  use_behavioral_HDL=off  hw_selection=Fabric  pipelined=off  block_type=addsub
  trotreal : xbsIndex_r4/AddSub  mode=Addition  use_carryin=off  use_carryout=off  en=off  latency=1  precision=User Defined  arith_type="Signed  (2's comp)"  n_bits=16  bin_pt=14  quantization=Truncate  overflow=Wrap  dbl_ovrd=off  use_behavioral_HDL=off  hw_selection=Fabric  pipelined=off  block_type=addsub
  Qt : Outport
  It : Outport  Port=2
  vld_out : Outport  Port=3
  wires:
  Q/1 -> trotimag/2
  trot_yoffset/1 -> trotimag/1
  I/1 -> trotreal/1
  trot_xoffset/1 -> trotreal/2
  trotreal/1 -> It/1
  trotimag/1 -> Qt/1
  Delay/1 -> vld_out/1
  vld_in/1 -> Delay/1

== system qdrdacsim/FRD/flrampfsmoutst ==
  out_reg : Inport
  assert_reg : xbsIndex_r4/Assert  assert_type=on  type_source=Explicitly  gui_display_data_type=Fixed-point  arith_type=Unsigned  n_bits=4  bin_pt=0  preci_type=Single  exp_width=8  frac_width=24  assert_rate=off  rate_source=Explicitly  period=1  output_port=on  block_type=assert
  cast_gw : xbsIndex_r4/Convert  gui_display_data_type=Fixed-point  arith_type=Unsigned  n_bits=32  bin_pt=0  float_type=Single  exp_bits=8  fraction_bits=24  quantization=Truncate  overflow=Wrap  en=off  latency=0  dbl_ovrd=off  pipeline=off  block_type=convert
  io_delay : xbsIndex_r4/Delay  rst=off  infoeditControl=Selection of Reset will increase slice count due to use of real FFs and instead of SRLs  en=off  latency=0  dbl_ovrd=off  reg_retiming=on  block_type=delay
  qdrdac_FRD_flrampfsmoutst_user_data_in : xbsIndex_r4/Gateway Out  inherit_from_input=off  hdl_port=on  timing_constraint=None  locs_specified=off  LOCs={}  UseAsDAC=off  DACChannel='1'  block_type=gatewayout
  reint1 : xbsIndex_r4/Reinterpret  force_arith_type=on  arith_type=Unsigned  force_bin_pt=on  bin_pt=0  block_type=reinterpret
  sim_out : Outport
  wires:
  io_delay/1 -> cast_gw/1
  cast_gw/1 -> qdrdac_FRD_flrampfsmoutst_user_data_in/1
  qdrdac_FRD_flrampfsmoutst_user_data_in/1 -> sim_out/1
  out_reg/1 -> assert_reg/1
  assert_reg/1 -> reint1/1
  reint1/1 -> io_delay/1

== system qdrdacsim/FRD/flrampfsmst ==
  out_reg : Inport
  assert_reg : xbsIndex_r4/Assert  assert_type=on  type_source=Explicitly  gui_display_data_type=Fixed-point  arith_type=Unsigned  n_bits=4  bin_pt=0  preci_type=Single  exp_width=8  frac_width=24  assert_rate=off  rate_source=Explicitly  period=1  output_port=on  block_type=assert
  cast_gw : xbsIndex_r4/Convert  gui_display_data_type=Fixed-point  arith_type=Unsigned  n_bits=32  bin_pt=0  float_type=Single  exp_bits=8  fraction_bits=24  quantization=Truncate  overflow=Wrap  en=off  latency=0  dbl_ovrd=off  pipeline=off  block_type=convert
  io_delay : xbsIndex_r4/Delay  rst=off  infoeditControl=Selection of Reset will increase slice count due to use of real FFs and instead of SRLs  en=off  latency=0  dbl_ovrd=off  reg_retiming=on  block_type=delay
  qdrdac_FRD_flrampfsmst_user_data_in : xbsIndex_r4/Gateway Out  inherit_from_input=off  hdl_port=on  timing_constraint=None  locs_specified=off  LOCs={}  UseAsDAC=off  DACChannel='1'  block_type=gatewayout
  reint1 : xbsIndex_r4/Reinterpret  force_arith_type=on  arith_type=Unsigned  force_bin_pt=on  bin_pt=0  block_type=reinterpret
  sim_out : Outport
  wires:
  io_delay/1 -> cast_gw/1
  cast_gw/1 -> qdrdac_FRD_flrampfsmst_user_data_in/1
  qdrdac_FRD_flrampfsmst_user_data_in/1 -> sim_out/1
  out_reg/1 -> assert_reg/1
  assert_reg/1 -> reint1/1
  reint1/1 -> io_delay/1
